simulink model "maglev_nonlinear"  (R2020b)
settings: Solver=VariableStepAuto  StartTime=0.0  StopTime=10.0  RelTol=1e-3
libraries: vrlib x2, pid_lib x1
settings Model: Creator=ApriZon  LastModifiedBy=ApriZon

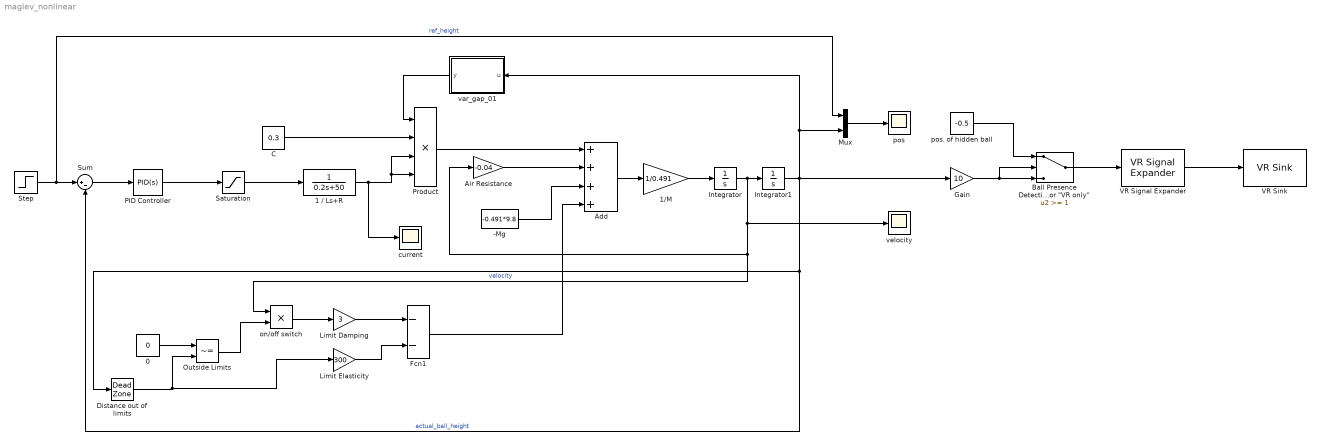
== system maglev_nonlinear ==
  -Mg : Constant  Value=-0.491*9.8
  0 : Constant  Value=0
  1 / Ls+R : TransferFcn  Denominator=[0.2 50]
  1/M : Gain  Gain=1/0.491
  Add : Sum  Inputs=++++
  Air Resistance : Gain  Gain=-0.04  OutDataTypeStr=double
  "Ball Presence Detection Value > Threshold = Ball Not Present 1 for \"VR only\"" : Switch  Threshold=1  ZeroCross=off  InputSameDT=on
  C : Constant  Value=0.3
  Distance out of limits : DeadZone  LowerValue=0.0002  UpperValue=0.0998  ZeroCross=off  SaturateOnIntegerOverflow=on
  Fcn1 : Sum  Inputs=--  InputSameDT=on  OutDataTypeStr=double  SaturateOnIntegerOverflow=on
  Gain : Gain  Gain=10
  Integrator : Integrator  ZeroCross=off
  Integrator1 : Integrator  InitialCondition=0.0001  LimitOutput=on  UpperSaturationLimit=0.1  LowerSaturationLimit=0  ZeroCross=off
  Limit Damping : Gain  Gain=3  OutDataTypeStr=double  SaturateOnIntegerOverflow=on  ParamDataTypeStr=Inherit: Same as input
  Limit Elasticity : Gain  Gain=300  OutDataTypeStr=double  SaturateOnIntegerOverflow=on  ParamDataTypeStr=Inherit: Same as input
  Mux : Mux  Inputs=2
  Outside Limits : RelationalOperator  Operator=~=  ZeroCross=off  RndMeth=Nearest  InputSameDT=on
  PID Controller : pid_lib/PID Controller  Controller=PID  Form=Parallel  TimeDomain=Continuous-time  UseExternalTs=off  SampleTime=-1  IntegratorMethod=Forward Euler  FilterMethod=Forward Euler  ControllerParametersSource=internal  P=1600  I=2634  D=244  UseFilter=on  N=100  TunerSelectOption=Transfer Function Based (PID Tuner App)  InitialConditionSource=internal  InitialConditionForIntegrator=0  InitialConditionForFilter=0  DifferentiatorICPrevScaledInput=0  ExternalReset=none  TrackingMode=off  Kt=1  LimitOutput=off  SatLimitsSource=internal  UpperSaturationLimit=inf  LowerSaturationLimit=-inf  LinearizeAsGain=on  AntiWindupMode=none  Kb=1  POutMin=[]  POutMax=[]  IOutMin=[]  IOutMax=[]  DOutMin=[]  DOutMax=[]  NOutMin=[]  NOutMax=[]  SumOutMin=[]  SumOutMax=[]  SaturationOutMin=[]  SaturationOutMax=[]  PParamMin=[]  PParamMax=[]  IParamMin=[]  IParamMax=[]  DParamMin=[]  DParamMax=[]  NParamMin=[]  NParamMax=[]  KbParamMin=[]  KbParamMax=[]  KtParamMin=[]  KtParamMax=[]  KbOutMin=[]  KbOutMax=[]  KtOutMin=[]  KtOutMax=[]  IntegratorOutMin=[]  IntegratorOutMax=[]  FilterOutMin=[]  FilterOutMax=[]  SumI1OutMin=[]  SumI1OutMax=[]  SumI2OutMin=[]  SumI2OutMax=[]  SumI3OutMin=[]  SumI3OutMax=[]  SumI4OutMin=[]  SumI4OutMax=[]  SumDOutMin=[]  SumDOutMax=[]  DifferentiatorOutMin=[]  DifferentiatorOutMax=[]  FilterDiffOutCoefMin=[]  FilterDiffOutCoefMax=[]  ReciprocalOutMin=[]  ReciprocalOutMax=[]  SumDenOutMin=[]  SumDenOutMax=[]  SumNumOutMin=[]  SumNumOutMax=[]  DivideOutMin=[]  DivideOutMax=[]  UdiffTsProdOutMin=[]  UdiffTsProdOutMax=[]  NTsProdOutMin=[]  NTsProdOutMax=[]  UintegralTsProdOutMin=[]  UintegralTsProdOutMax=[]  UngainTsProdOutMin=[]  UngainTsProdOutMax=[]  IntegratorContinuousStateAttributes=''  IntegratorStateMustResolveToSignalObject=off  IntegratorRTWStateStorageClass=Auto  FilterContinuousStateAttributes=''  FilterStateMustResolveToSignalObject=off  FilterRTWStateStorageClass=Auto  ParallelPVariant=InternalParameters  IdealPVariant=Disabled  IVariant=InternalParameters  DVariant=InternalParameters  IntegratorVariant=Continuous  SatVariant=Disabled  AWVariant=Passthrough  PCopyVariant=Disabled  TRVariant=Disabled  FdbkBlocksVariant=Forward  IdealPFdbkVariant=Disabled  SatFdbkVariant=Disabled  DerivativeFilterVariant=ContFilter  NVariant=InternalParameters  NCopyVariant=Disabled  FilterICVariant=InternalICsFilter  IntegratorICVariant=InternalICs  ExternalResetVariant=Disabled  TRSumVariant=Passthrough  SumFdbkVariant=Disabled  SumVariant=Sum_PID  TsampFilterVariant=InternalTs  TsampNgainVariant=Passthrough  TsampIntegralVariant=Passthrough  ExternalSaturationOutDataTypeStr=Inherit: Same as second input
  Product : Product  Inputs=4  OutDataTypeStr=double
  Saturation : Saturate  UpperLimit=200  LowerLimit=0  ZeroCross=off
  Step : Step  Time=0  After=0.08  SampleTime=0  ZeroCross=off
  Sum : Sum  Inputs=|+-
  VR Signal Expander : vrlib/VR Signal Expander  outwidth=3  outidx=[2]
  VR Sink : vrlib/VR Sink  InstantiateOnLoad=on  SampleTime=0.02  ViewEnable=on  RemoteChange=off  RemoteView=off  FieldsWritten=Ball.translation.3.1.1.double  WorldFileName=maglev.wrl  WorldDescription=VR Magnetic Levitation Model  AutoView=off  VideoDimensions=[]  AllowVariableSize=off
  current : Scope
  on/off switch : Product  OutDataTypeStr=double  SaturateOnIntegerOverflow=on
  pos : Scope
  pos. of hidden ball : Constant  Value=-0.5
  var_gap_01 : MATLAB Function  TreatAsAtomicUnit=on
  velocity : Scope
  wires:
  Step/1 -> Mux/1, Sum/1  "ref_height"
  Sum/1 -> PID Controller/1
  Saturation/1 -> 1 / Ls+R/1
  1 / Ls+R/1 -> current/1, Product/4, Product/3
  C/1 -> Product/2
  var_gap_01/1(y) -> Product/1
  Product/1 -> Add/1
  -Mg/1 -> Add/3
  Air Resistance/1 -> Add/2
  Add/1 -> 1/M/1
  1/M/1 -> Integrator/1
  Integrator/1 -> velocity/1, on/off switch/1, Air Resistance/1, Integrator1/1  "velocity"
  Integrator1/1 -> Gain/1, Mux/2, var_gap_01/1(u), Distance out of limits/1, Sum/2  "actual_ball_height"
  Limit Damping/1 -> Fcn1/1
  Limit Elasticity/1 -> Fcn1/2
  on/off switch/1 -> Limit Damping/1
  Outside Limits/1 -> on/off switch/2
  0/1 -> Outside Limits/1
  PID Controller/1 -> Saturation/1
  Mux/1 -> pos/1
  Gain/1 -> "Ball Presence Detection Value > Threshold = Ball Not Present 1 for \"VR only\""/2, "Ball Presence Detection Value > Threshold = Ball Not Present 1 for \"VR only\""/3
  pos. of hidden ball/1 -> "Ball Presence Detection Value > Threshold = Ball Not Present 1 for \"VR only\""/1
  "Ball Presence Detection Value > Threshold = Ball Not Present 1 for \"VR only\""/1 -> VR Signal Expander/1
  VR Signal Expander/1 -> VR Sink/1
  Fcn1/1 -> Add/4
  Distance out of limits/1 -> Limit Elasticity/1, Outside Limits/2

== matlab function maglev_nonlinear/var_gap_01 ==
  data: u input; y output
function y = fcn(u)
%#codegen

y = 1 / (0.1001 - u);
